simulink subsystem "caravann"  (R2023a)
settings: Solver=VariableStepAuto  StartTime=0.0  StopTime=10.0  RelTol=1e-3
values from neighbouring files (symbols this model uses):
  aeroDragCoeff = 0.18    [run_model.m]
  airDensity = 1.293    [run_model.m]
  frontArea = 3    [run_model.m]
  gravity = 9.81    [run_model.m]
  massSPC = massBatt + massCaravan + massStorage + nTires * massTire    (= 975.625)    [run_model.m]
  rollingResistCoeff = 0.008    [run_model.m]
undefined symbols (not defined in the file or in its folder): magnitude
libraries: fl_lib x5, nesl_utility x5, simulink x1
settings Model: Creator=sandu  LastModifiedBy=sandu

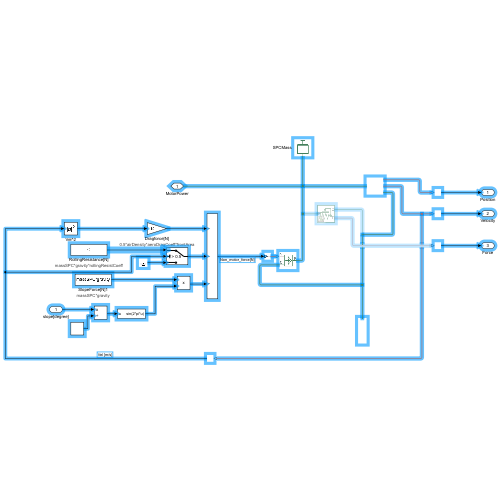
[thumbnail: Simulink's stored preview of the top-level diagram]
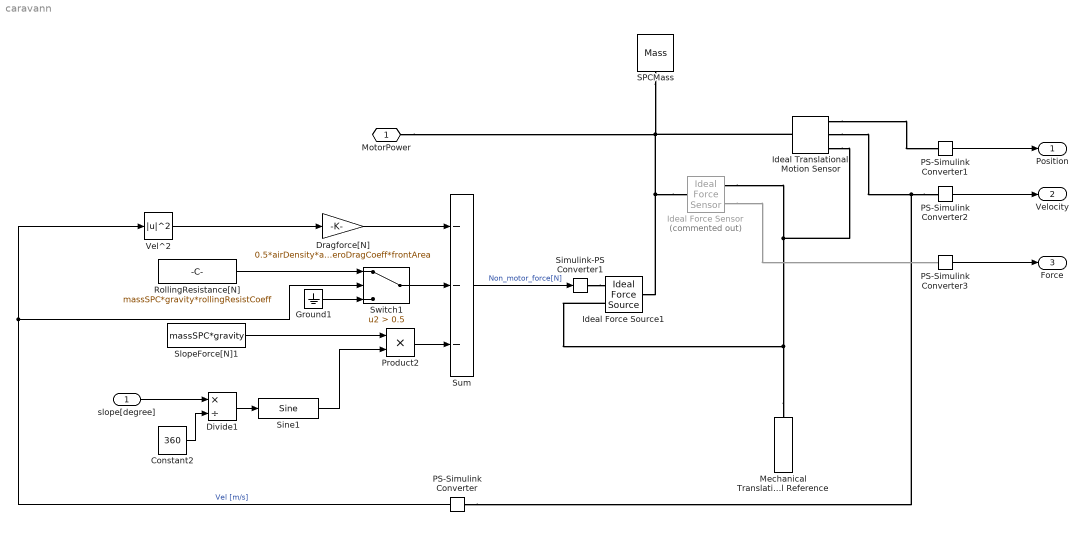
== system caravann ==
  slope[degree] : Inport
  Constant2 : Constant  Value=360
  Divide1 : Product  Inputs=*/
  Dragforce[N] : Gain  Gain=0.5*airDensity*aeroDragCoeff*frontArea
      settings: AttributesFormatString=%<Gain>
  Ground1 : Ground
  Ideal Force Sensor : fl_lib/Mechanical/Mechanical Sensors/Ideal Force Sensor  Commented=on
  Ideal Force Source1 : fl_lib/Mechanical/Mechanical Sources/Ideal Force Source
  Ideal Translational Motion Sensor : fl_lib/Mechanical/Mechanical Sensors/Ideal Translational Motion Sensor  reference=foundation.enum.MeasurementReference.difference  acceleration_port=false  velocity_port=true  position_port=true  offset=0 m
  Mechanical Translational Reference : fl_lib/Mechanical/Translational Elements/Mechanical Translational Reference
  PS-Simulink Converter{,1..3} (4 alike) : nesl_utility/PS-Simulink Converter  PhysicalDomain=network_engine_domain  SubClassName=ps_output  LeftPortType=input  RightPortType=output  PseudoPeriodic=off  Frequencies=[]  VectorFormat=inherit  Unit=inherit  AffineConversion=off
  Product2 : Product
  RollingResistance[N] : Constant  Value=massSPC*gravity*rollingResistCoeff
      settings: AttributesFormatString=%<Value>
  SPCMass : fl_lib/Mechanical/Translational Elements/Mass  mass=inertialMassSPC kg  num_ports=foundation.enum.numPorts2.one  v_specify=off  v_priority=High  v=1 m/s  v_nominal_specify=off  v_nominal_unit=m/s  v_nominal_value=1  f_specify=off  f_priority=None  f=0 N  f_nominal_specify=off  f_nominal_unit=N  f_nominal_value=1
  Simulink-PS Converter1 : nesl_utility/Simulink-PS Converter  PhysicalDomain=network_engine_domain  SubClassName=ps_input  LeftPortType=input  RightPortType=output  PseudoPeriodic=off  Frequencies=[]  NoiseDistribution=none  NoiseParameters=[]  Unit=1  AffineConversion=off  FilteringAndDerivatives=provide  SimscapeFilterOrder=1  InputFilterTimeConstant=0.001  UdotUserProvided=0
  Sine1 : simulink/Lookup Tables/Sine  Formula=sin(2*pi*u)  NumDataPoints=(2^5)+1  OutputWordLength=16  InternalRulePriority=Speed
  SlopeForce[N]1 : Constant  Value=massSPC*gravity
      settings: AttributesFormatString=%<Value>
  Sum : Sum  Inputs=---
  Switch1 : Switch  Criteria=u2 > Threshold  Threshold=0.5  SaturateOnIntegerOverflow=off  InputSameDT=off
  Vel^2 : Math  Operator=magnitude^2  SignedPower=on
  MotorPower : PMIOPort  Side=Left
  Position : Outport
  Velocity : Outport  Port=2
  Force : Outport  Port=3
  wires:
  PS-Simulink Converter3/1 -> Force/1
  PS-Simulink Converter1/1 -> Position/1
  Divide1/1 -> Sine1/1
  PS-Simulink Converter/1 -> Vel^2/1, Switch1/2  "Vel [m/s]"
  Ground1/1 -> Switch1/3
  Product2/1 -> Sum/3
  Sine1/1 -> Product2/2
  PS-Simulink Converter2/1 -> Velocity/1
  Dragforce[N]/1 -> Sum/1
  Constant2/1 -> Divide1/2
  Vel^2/1 -> Dragforce[N]/1
  Sum/1 -> Simulink-PS Converter1/1  "Non_motor_force[N]"
  SlopeForce[N]1/1 -> Product2/1
  slope[degree]/1 -> Divide1/1
  Switch1/1 -> Sum/2
  RollingResistance[N]/1 -> Switch1/1
  connections:
  Ideal Force Sensor/LConn1 -- SPCMass/LConn1 -- MotorPower/RConn1 -- Ideal Translational Motion Sensor/LConn1 -- Ideal Force Source1/LConn1
  Mechanical Translational Reference/LConn1 -- Ideal Force Source1/RConn2 -- Ideal Translational Motion Sensor/RConn1 -- Ideal Force Sensor/RConn1
  PS-Simulink Converter2/LConn1 -- Ideal Translational Motion Sensor/RConn2 -- PS-Simulink Converter/LConn1
  Ideal Translational Motion Sensor/RConn3 -- PS-Simulink Converter1/LConn1
  Ideal Force Sensor/RConn2 -- PS-Simulink Converter3/LConn1
  Simulink-PS Converter1/RConn1 -- Ideal Force Source1/RConn1
